simulink model "L4OLARUa"  (R2020b)
settings: Solver=VariableStepAuto  StartTime=0.0  StopTime=15000  RelTol=1e-3
values from neighbouring files (symbols this model uses):
  kc = 125    [paramsL4.m]
  kE = 1000    [paramsL4.m]
  kp = 500    [paramsL4.m]
  Tc = 300    [paramsL4.m]
  Tp = 60    [paramsL4.m]
settings Model: Creator=olaru  LastModifiedBy=olaru

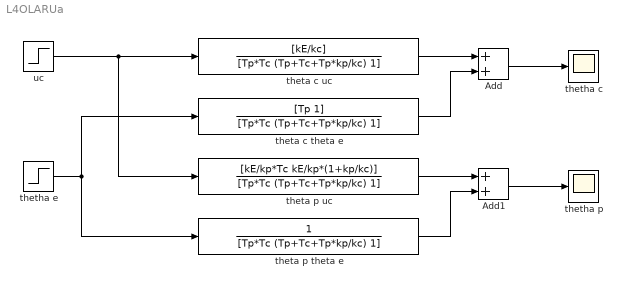
== system L4OLARUa ==
  Add : Sum
  Add1 : Sum
  theta c theta e : TransferFcn  Numerator=[Tp 1]  Denominator=[Tp*Tc (Tp+Tc+Tp*kp/kc) 1]
  theta c uc : TransferFcn  Numerator=[kE/kc]  Denominator=[Tp*Tc (Tp+Tc+Tp*kp/kc) 1]
  theta p theta e : TransferFcn  Denominator=[Tp*Tc (Tp+Tc+Tp*kp/kc) 1]
  theta p uc : TransferFcn  Numerator=[kE/kp*Tc kE/kp*(1+kp/kc)]  Denominator=[Tp*Tc (Tp+Tc+Tp*kp/kc) 1]
  thetha c : Scope
  thetha e : Step  Time=5000  After=-10  SampleTime=0
  thetha p : Scope
  uc : Step  Time=0  After=2.5  SampleTime=0
  wires:
  thetha e/1 -> theta p theta e/1, theta c theta e/1
  uc/1 -> theta p uc/1, theta c uc/1
  theta c theta e/1 -> Add/2
  theta c uc/1 -> Add/1
  theta p uc/1 -> Add1/1
  theta p theta e/1 -> Add1/2
  Add1/1 -> thetha p/1
  Add/1 -> thetha c/1
